simulink model "simulink_model"  (R2016b)
settings: Solver=ode45  StartTime=0.0  StopTime=200  RelTol=1e-3  EnableMultiTasking=on
libraries: fuzblock x1
settings Model: Creator=stefk  LastModifiedBy=stefkon
settings DataIOCC: LimitDataPoints=on  SaveFormat=Array
settings OptimizationCC: LifeSpan=inf
settings DebuggingCC: SFUnexpectedBacktrackingDiag=warning  SFNoUnconditionalDefaultTransitionDiag=warning  SFExecutionAtInitializationDiag=none
settings HardwareCC: ProdBitPerPointer=32  ProdBitPerSizeT=32  ProdBitPerPtrDiffT=32  ProdLargestAtomicFloat=None  ProdIntDivRoundTo=Undefined  ProdEndianess=Unspecified  ProdWordSize=32  ProdHWDeviceType=32-bit Generic
settings ModelReferenceCC: PropagateSignalLabelsOutOfModel=off
settings GRTTargetCC: TargetLangStandard=C89/C90 (ANSI)  GeneratePreprocessorConditionals=Disable all
settings ConfigComp: CovMetricSettings=dw  CovHtmlReporting=on  CovSaveCumulativeToWorkspaceVar=on  CovSaveSingleToWorkspaceVar=on  CovExternalEMLEnable=off

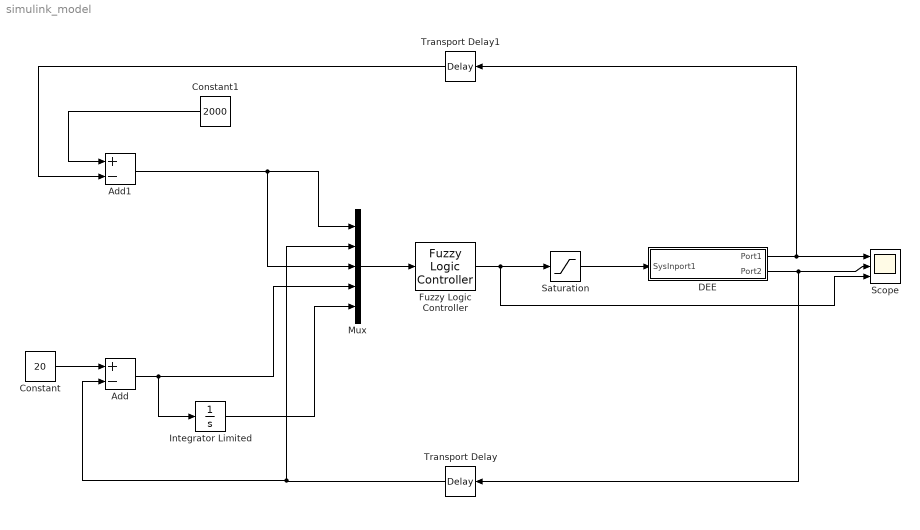
== system simulink_model ==
  Add : Sum  Inputs=+-
  Add1 : Sum  Inputs=+-
  Constant : Constant  Value=20
  Constant1 : Constant  Value=2000
  DEE : Subsystem  mask(Differential Equation Editor (DEE)){}
      settings: OpenFcn=diffeqed
      mask Display: disp('train_model')
  Fuzzy Logic Controller : fuzblock/Fuzzy Logic  Controller  fis='train_fuzzy.fis'
  Integrator Limited : Integrator  LimitOutput=on  UpperSaturationLimit=20  LowerSaturationLimit=-20
  Mux : Mux  Inputs=5
  Saturation : Saturate  UpperLimit=20  LowerLimit=-20
  Scope : Scope  NumInputPorts=3
  Transport Delay : TransportDelay
  Transport Delay1 : TransportDelay
  wires:
  Mux/1 -> Fuzzy Logic Controller/1
  Constant/1 -> Add/1
  Add/1 -> Integrator Limited/1, Mux/4
  Constant1/1 -> Add1/1
  Add1/1 -> Mux/3, Mux/1
  DEE/1(Port1) -> Transport Delay1/1, Scope/1
  Integrator Limited/1 -> Mux/5
  DEE/2(Port2) -> Transport Delay/1, Scope/2
  Transport Delay/1 -> Mux/2, Add/2
  Transport Delay1/1 -> Add1/2
  Fuzzy Logic Controller/1 -> Saturation/1, Scope/3
  Saturation/1 -> DEE/1(SysInport1)

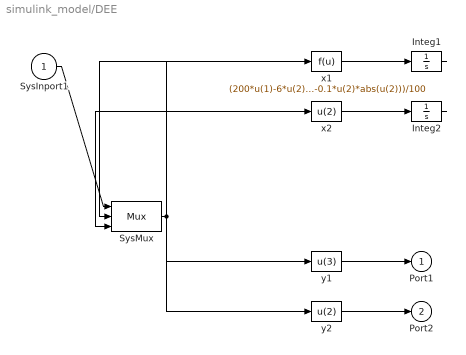
== system simulink_model/DEE ==
  SysInport1 : Inport
  Integ1 : Integrator
  Integ2 : Integrator
  SysMux : Mux  Inputs=3
  x1 : Fcn  Expr=(200*u(1)-6*u(2)-0.1*u(2)*abs(u(2)))/100
  x2 : Fcn  Expr=u(2)
  y1 : Fcn  Expr=u(3)
  y2 : Fcn  Expr=u(2)
  Port1 : Outport
  Port2 : Outport  Port=2
  wires:
  SysInport1/1 -> SysMux/1
  SysMux/1 -> x1/1, x2/1, y1/1, y2/1
  x1/1 -> Integ1/1
  Integ1/1 -> SysMux/2
  x2/1 -> Integ2/1
  Integ2/1 -> SysMux/3
  y1/1 -> Port1/1
  y2/1 -> Port2/1
